simulink model "MBD_WEEK2_QN3"  (R2020b)
settings: Solver=VariableStepAuto  StartTime=0.0  StopTime=10  RelTol=1e-3
values from neighbouring files (symbols this model uses):
  b = 50    [Variables.m]
  m = 1000    [Variables.m]
settings Model: DataDictionary=cruise_control_data.sldd  OrderedModelArguments=off  Creator=dell  LastModifiedBy=dell

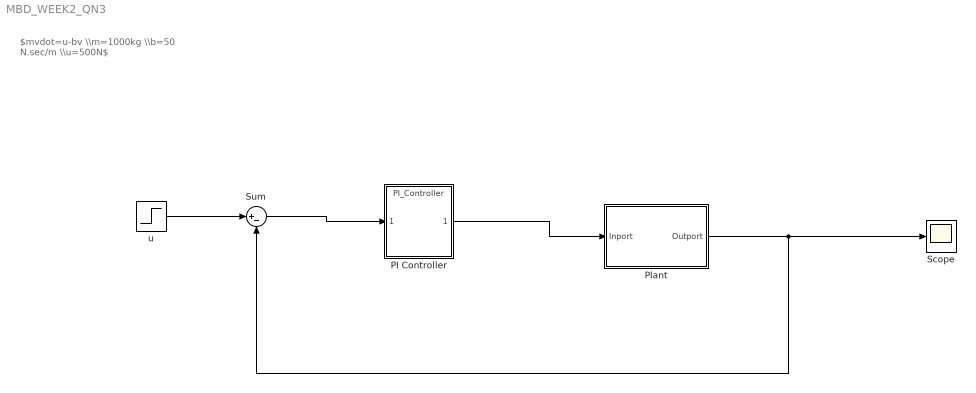
== system MBD_WEEK2_QN3 ==
  note: $mvdot=u-bv \\m=1000kg \\b=50 N.sec/m \\u=500N$
  PI Controller : ModelReference  ModelNameDialog=PI_Controller  SimulationMode=Normal  ModelReferenceVersion=1.14
  Plant : Subsystem
  Scope : Scope
  Sum : Sum  Inputs=|+-
  u : Step  Time=0  After=10  SampleTime=0
  wires:
  u/1 -> Sum/1
  Plant/1(Outport) -> Sum/2, Scope/1
  PI Controller/1 -> Plant/1(Inport)
  Sum/1 -> PI Controller/1

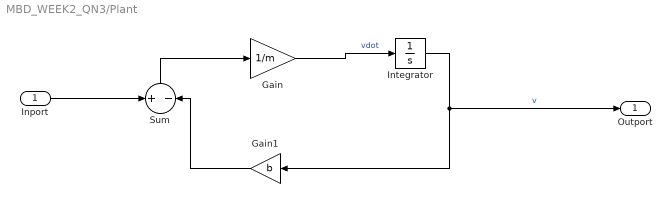
== system MBD_WEEK2_QN3/Plant ==
  Inport : Inport
  Gain : Gain  Gain=1/m
  Gain1 : Gain  Gain=b
  Integrator : Integrator
  Sum : Sum  Inputs=+-
  Outport : Outport
  wires:
  Integrator/1 -> Outport/1, Gain1/1  "v"
  Sum/1 -> Gain/1
  Gain/1 -> Integrator/1  "vdot"
  Inport/1 -> Sum/1
  Gain1/1 -> Sum/2
